simulink model "model_main5"  (R2023b)
settings: Solver=ode4  StartTime=0.0  StopTime=1000  FixedStep=dt  RelTol=1e-3
InitFcn:
  | model_init
values from neighbouring files (symbols this model uses):
  dt = 0.01    [model_init.m]
  Iws = diag([1 1 1 1])*0.2274    [model_init.m]
  m_tot = 3300    [model_init.m]
  norm_Ib = diag(diag(SC_Ib) / norm(diag(SC_Ib)))    [model_init.m]
  Omega1_init = 2000*rpm2rad    (= 209.439510239)    [model_init.m]
  Omega2_init = 2000*rpm2rad    (= 209.439510239)    [model_init.m]
  Omega3_init = 2000*rpm2rad    (= 209.439510239)    [model_init.m]
  Omega4_init = 2000*rpm2rad    (= 209.439510239)    [model_init.m]
  Omega_ref = [1000 1000 1000 1000]*rpm2rad    [model_init.m]
  port_offset = [7.196; 0 ; 0.618]    [model_init.m]
  qb0 = angle2quat(ag0(1),ag0(2),ag0(3),'ZYX')'    [model_init.m]
  rad2rpm = 1/rpm2rad    (= 9.54929658551)    [model_init.m]
  RCS_F = 1.0    (= 1)    [model_init.m]
  RCS_Pos = [RCS1_POS , RCS2_POS , RCS3_POS , RCS4_POS ,            RCS5_POS , RCS6_POS , RCS7_POS , RCS8_POS ,            RCS9_POS , RCS10_POS, RCS11_POS, RCS12_POS,            RCS13_POS, RCS14_POS, RCS15_POS, RCS16_POS]    [model_init.m]
  RCS_PWM_Freq = 0.1    [model_init.m]
  RCS_Sampling_time = 0.01    [model_init.m]
  RCS_THR_vec = [RCS1_THR , RCS2_THR , RCS3_THR , RCS4_THR,                 RCS5_THR , RCS6_THR , RCS7_THR , RCS8_THR,                 RCS9_THR , RCS10_THR, RCS11_THR, RCS12_THR,                 RCS13_THR, RCS14_THR, RCS15_THR, RCS16_THR]    [model_init.m]
  REL_port_POS_I_0 = REL_TS_POS_I_0 - quat2rotm(qb0') * port_offset    [model_init.m]
  REL_port_VEL_I_0 = REL_TS_VEL_I_0 - quat2rotm(qb0') * cross(wb0,port_offset)    [model_init.m]
  REL_TS_POS_I_0 = TS_pos0 - SC_pos0    [model_init.m]
  REL_TS_VEL_I_0 = TS_vel0 - SC_vel0    [model_init.m]
  RW_As = [RW1_Axis,RW2_Axis,RW3_Axis,RW4_Axis]    [model_init.m]
  RW_Max_Speed = 4200*rpm2rad    (= 439.822971503)    [model_init.m]
  RW_t_max = 0.5    [model_init.m]
  SC_Ib = [1843.56  -0.0019  -803.89 ... (first row only)    [model_init.m]
  SC_state0 = kepel_statvec (SC_Kepler)    [model_init.m]
  TS_Ib = diag([1 1 1])    [model_init.m]
  TS_qb0 = angle2quat(deg2rad(0),deg2rad(0),deg2rad(0),'ZYX')'    [model_init.m]
  TS_state0 = kepel_statvec (TS_Kepler)    [model_init.m]
  TS_wb0 = deg2rad([0 0 0]')    [model_init.m]
  wb0 = deg2rad([-0.3 -0.1 0.2])'    [model_init.m]
undefined symbols (not defined in the file or in its folder): RCS_F_vec, RCS_pos, SS_Total_Mass, TC_Kepler
libraries: simulink x16, simulink_extras x16, aerolibutil x9, sharedtransform x8
(part 2 of 3)

== system model_main5/PWPFM/Subsystem2 ==
  In1 : Inport
  Constant : Constant  Value=0
  Constant1 : Constant
  PWPFM_Filter2 : TransferFcn  Numerator=1  Denominator=[0.275 1]
  Schmitt_Trigger1 : Relay  OnSwitchValue=0.127  OffSwitchValue=-0.127
  Sum_PWPFM1 : Sum  Inputs=|+-
  Switch : Switch  Criteria=u2 > Threshold  Threshold=0.25  SaturateOnIntegerOverflow=off  InputSameDT=off
  Switch2 : Switch  Criteria=u2 > Threshold  Threshold=1  SaturateOnIntegerOverflow=off  InputSameDT=off
  F_gated : Outport
  wires:
  In1/1 -> Switch/2, Switch/1
  Constant/1 -> Switch/3
  Switch/1 -> Switch2/2, Switch2/3
  Constant1/1 -> Switch2/1
  Switch2/1 -> Sum_PWPFM1/1
  Schmitt_Trigger1/1 -> PWPFM_Filter2/1, F_gated/1
  Sum_PWPFM1/1 -> Schmitt_Trigger1/1
  PWPFM_Filter2/1 -> Sum_PWPFM1/2

== system model_main5/PWPFM/Subsystem3 ==
  In1 : Inport
  Constant : Constant  Value=0
  Constant1 : Constant
  PWPFM_Filter2 : TransferFcn  Numerator=1  Denominator=[0.275 1]
  Schmitt_Trigger1 : Relay  OnSwitchValue=0.127  OffSwitchValue=-0.127
  Sum_PWPFM1 : Sum  Inputs=|+-
  Switch : Switch  Criteria=u2 > Threshold  Threshold=0.25  SaturateOnIntegerOverflow=off  InputSameDT=off
  Switch2 : Switch  Criteria=u2 > Threshold  Threshold=1  SaturateOnIntegerOverflow=off  InputSameDT=off
  F_gated : Outport
  wires:
  PWPFM_Filter2/1 -> Sum_PWPFM1/2
  Sum_PWPFM1/1 -> Schmitt_Trigger1/1
  Schmitt_Trigger1/1 -> F_gated/1, PWPFM_Filter2/1
  Switch2/1 -> Sum_PWPFM1/1
  Constant1/1 -> Switch2/1
  Switch/1 -> Switch2/3, Switch2/2
  Constant/1 -> Switch/3
  In1/1 -> Switch/1, Switch/2

== system model_main5/PWPFM/Subsystem4 ==
  In1 : Inport
  Constant : Constant  Value=0
  Constant1 : Constant
  PWPFM_Filter2 : TransferFcn  Numerator=1  Denominator=[0.275 1]
  Schmitt_Trigger1 : Relay  OnSwitchValue=0.127  OffSwitchValue=-0.127
  Sum_PWPFM1 : Sum  Inputs=|+-
  Switch : Switch  Criteria=u2 > Threshold  Threshold=0.25  SaturateOnIntegerOverflow=off  InputSameDT=off
  Switch2 : Switch  Criteria=u2 > Threshold  Threshold=1  SaturateOnIntegerOverflow=off  InputSameDT=off
  F_gated : Outport
  wires:
  In1/1 -> Switch/2, Switch/1
  Constant/1 -> Switch/3
  Switch/1 -> Switch2/2, Switch2/3
  Constant1/1 -> Switch2/1
  Switch2/1 -> Sum_PWPFM1/1
  Schmitt_Trigger1/1 -> PWPFM_Filter2/1, F_gated/1
  Sum_PWPFM1/1 -> Schmitt_Trigger1/1
  PWPFM_Filter2/1 -> Sum_PWPFM1/2

== system model_main5/PWPFM/Subsystem5 ==
  In1 : Inport
  Constant : Constant  Value=0
  Constant1 : Constant
  PWPFM_Filter2 : TransferFcn  Numerator=1  Denominator=[0.275 1]
  Schmitt_Trigger1 : Relay  OnSwitchValue=0.127  OffSwitchValue=-0.127
  Sum_PWPFM1 : Sum  Inputs=|+-
  Switch : Switch  Criteria=u2 > Threshold  Threshold=0.25  SaturateOnIntegerOverflow=off  InputSameDT=off
  Switch2 : Switch  Criteria=u2 > Threshold  Threshold=1  SaturateOnIntegerOverflow=off  InputSameDT=off
  F_gated : Outport
  wires:
  PWPFM_Filter2/1 -> Sum_PWPFM1/2
  Sum_PWPFM1/1 -> Schmitt_Trigger1/1
  Schmitt_Trigger1/1 -> F_gated/1, PWPFM_Filter2/1
  Switch2/1 -> Sum_PWPFM1/1
  Constant1/1 -> Switch2/1
  Switch/1 -> Switch2/3, Switch2/2
  Constant/1 -> Switch/3
  In1/1 -> Switch/1, Switch/2

== system model_main5/PWPFM/Subsystem6 ==
  In1 : Inport
  Constant : Constant  Value=0
  Constant1 : Constant
  PWPFM_Filter2 : TransferFcn  Numerator=1  Denominator=[0.275 1]
  Schmitt_Trigger1 : Relay  OnSwitchValue=0.127  OffSwitchValue=-0.127
  Sum_PWPFM1 : Sum  Inputs=|+-
  Switch : Switch  Criteria=u2 > Threshold  Threshold=0.25  SaturateOnIntegerOverflow=off  InputSameDT=off
  Switch2 : Switch  Criteria=u2 > Threshold  Threshold=1  SaturateOnIntegerOverflow=off  InputSameDT=off
  F_gated : Outport
  wires:
  In1/1 -> Switch/2, Switch/1
  Constant/1 -> Switch/3
  Switch/1 -> Switch2/2, Switch2/3
  Constant1/1 -> Switch2/1
  Switch2/1 -> Sum_PWPFM1/1
  Schmitt_Trigger1/1 -> PWPFM_Filter2/1, F_gated/1
  Sum_PWPFM1/1 -> Schmitt_Trigger1/1
  PWPFM_Filter2/1 -> Sum_PWPFM1/2

== system model_main5/PWPFM/Subsystem7 ==
  In1 : Inport
  Constant : Constant  Value=0
  Constant1 : Constant
  PWPFM_Filter2 : TransferFcn  Numerator=1  Denominator=[0.275 1]
  Schmitt_Trigger1 : Relay  OnSwitchValue=0.127  OffSwitchValue=-0.127
  Sum_PWPFM1 : Sum  Inputs=|+-
  Switch : Switch  Criteria=u2 > Threshold  Threshold=0.25  SaturateOnIntegerOverflow=off  InputSameDT=off
  Switch2 : Switch  Criteria=u2 > Threshold  Threshold=1  SaturateOnIntegerOverflow=off  InputSameDT=off
  F_gated : Outport
  wires:
  In1/1 -> Switch/2, Switch/1
  Constant/1 -> Switch/3
  Switch/1 -> Switch2/2, Switch2/3
  Constant1/1 -> Switch2/1
  Switch2/1 -> Sum_PWPFM1/1
  Schmitt_Trigger1/1 -> PWPFM_Filter2/1, F_gated/1
  Sum_PWPFM1/1 -> Schmitt_Trigger1/1
  PWPFM_Filter2/1 -> Sum_PWPFM1/2

== system model_main5/PWPFM/Subsystem8 ==
  In1 : Inport
  Constant : Constant  Value=0
  Constant1 : Constant
  PWPFM_Filter2 : TransferFcn  Numerator=1  Denominator=[0.275 1]
  Schmitt_Trigger1 : Relay  OnSwitchValue=0.127  OffSwitchValue=-0.127
  Sum_PWPFM1 : Sum  Inputs=|+-
  Switch : Switch  Criteria=u2 > Threshold  Threshold=0.25  SaturateOnIntegerOverflow=off  InputSameDT=off
  Switch2 : Switch  Criteria=u2 > Threshold  Threshold=1  SaturateOnIntegerOverflow=off  InputSameDT=off
  F_gated : Outport
  wires:
  PWPFM_Filter2/1 -> Sum_PWPFM1/2
  Sum_PWPFM1/1 -> Schmitt_Trigger1/1
  Schmitt_Trigger1/1 -> F_gated/1, PWPFM_Filter2/1
  Switch2/1 -> Sum_PWPFM1/1
  Constant1/1 -> Switch2/1
  Switch/1 -> Switch2/3, Switch2/2
  Constant/1 -> Switch/3
  In1/1 -> Switch/1, Switch/2

== system model_main5/PWPFM/Subsystem9 ==
  In1 : Inport
  Constant : Constant  Value=0
  Constant1 : Constant
  PWPFM_Filter2 : TransferFcn  Numerator=1  Denominator=[0.275 1]
  Schmitt_Trigger1 : Relay  OnSwitchValue=0.127  OffSwitchValue=-0.127
  Sum_PWPFM1 : Sum  Inputs=|+-
  Switch : Switch  Criteria=u2 > Threshold  Threshold=0.25  SaturateOnIntegerOverflow=off  InputSameDT=off
  Switch2 : Switch  Criteria=u2 > Threshold  Threshold=1  SaturateOnIntegerOverflow=off  InputSameDT=off
  F_gated : Outport
  wires:
  In1/1 -> Switch/2, Switch/1
  Constant/1 -> Switch/3
  Switch/1 -> Switch2/2, Switch2/3
  Constant1/1 -> Switch2/1
  Switch2/1 -> Sum_PWPFM1/1
  Schmitt_Trigger1/1 -> PWPFM_Filter2/1, F_gated/1
  Sum_PWPFM1/1 -> Schmitt_Trigger1/1
  PWPFM_Filter2/1 -> Sum_PWPFM1/2

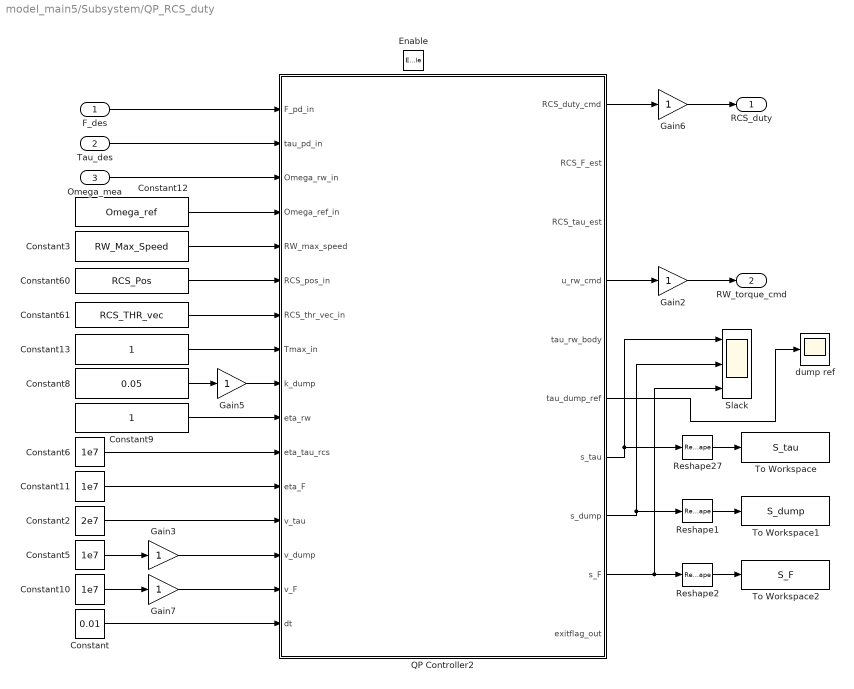
== system model_main5/Subsystem/QP_RCS_duty ==
  F_des : Inport
  Tau_des : Inport  Port=2
  Omega_mea : Inport  Port=3
  Enable : EnablePort
  Constant : Constant  Value=0.01
  Constant{5..6,10..11} (4 alike) : Constant  Value=1e7
  Constant12 : Constant  Value=Omega_ref
  Constant13 : Constant
  Constant2 : Constant  Value=2e7
  Constant3 : Constant  Value=RW_Max_Speed
  Constant60 : Constant  Value=RCS_Pos
  Constant61 : Constant  Value=RCS_THR_vec
  Constant8 : Constant  Value=0.05
  Constant9 : Constant
  Gain{2..3,5..7} (5 alike) : Gain
  QP Controller2 : MATLAB Function  TreatAsAtomicUnit=on
  Reshape1 : Reshape  OutputDimensionality=Row vector (2-D)
  Reshape2 : Reshape  OutputDimensionality=Row vector (2-D)
  Reshape27 : Reshape  OutputDimensionality=Row vector (2-D)
  Slack : Scope  NumInputPorts=3
  To Workspace : ToWorkspace  VariableName=S_tau  SampleTime=-1
  To Workspace1 : ToWorkspace  VariableName=S_dump  SampleTime=-1
  To Workspace2 : ToWorkspace  VariableName=S_F  SampleTime=-1
  dump ref : Scope
  RCS_duty : Outport
  RW_torque_cmd : Outport  Port=2
  wires:
  QP Controller2/4(u_rw_cmd) -> Gain2/1
  Tau_des/1 -> QP Controller2/2(tau_pd_in)
  Omega_mea/1 -> QP Controller2/3(Omega_rw_in)
  Constant3/1 -> QP Controller2/5(RW_max_speed)
  Constant2/1 -> QP Controller2/13(v_tau)
  Constant6/1 -> QP Controller2/11(eta_tau_rcs)
  Constant5/1 -> Gain3/1
  Constant/1 -> QP Controller2/16(dt)
  Gain2/1 -> RW_torque_cmd/1
  Gain3/1 -> QP Controller2/14(v_dump)
  Constant12/1 -> QP Controller2/4(Omega_ref_in)
  Constant8/1 -> Gain5/1
  Constant9/1 -> QP Controller2/10(eta_rw)
  Gain5/1 -> QP Controller2/9(k_dump)
  F_des/1 -> QP Controller2/1(F_pd_in)
  QP Controller2/1(RCS_duty_cmd) -> Gain6/1
  Gain6/1 -> RCS_duty/1
  Constant10/1 -> Gain7/1
  Gain7/1 -> QP Controller2/15(v_F)
  Constant11/1 -> QP Controller2/12(eta_F)
  QP Controller2/7(s_tau) -> Slack/1, Reshape27/1
  QP Controller2/8(s_dump) -> Reshape1/1, Slack/2
  QP Controller2/9(s_F) -> Reshape2/1, Slack/3
  Reshape27/1 -> To Workspace/1
  Reshape1/1 -> To Workspace1/1
  Reshape2/1 -> To Workspace2/1
  Constant61/1 -> QP Controller2/7(RCS_thr_vec_in)
  QP Controller2/6(tau_dump_ref) -> dump ref/1
  Constant13/1 -> QP Controller2/8(Tmax_in)
  Constant60/1 -> QP Controller2/6(RCS_pos_in)

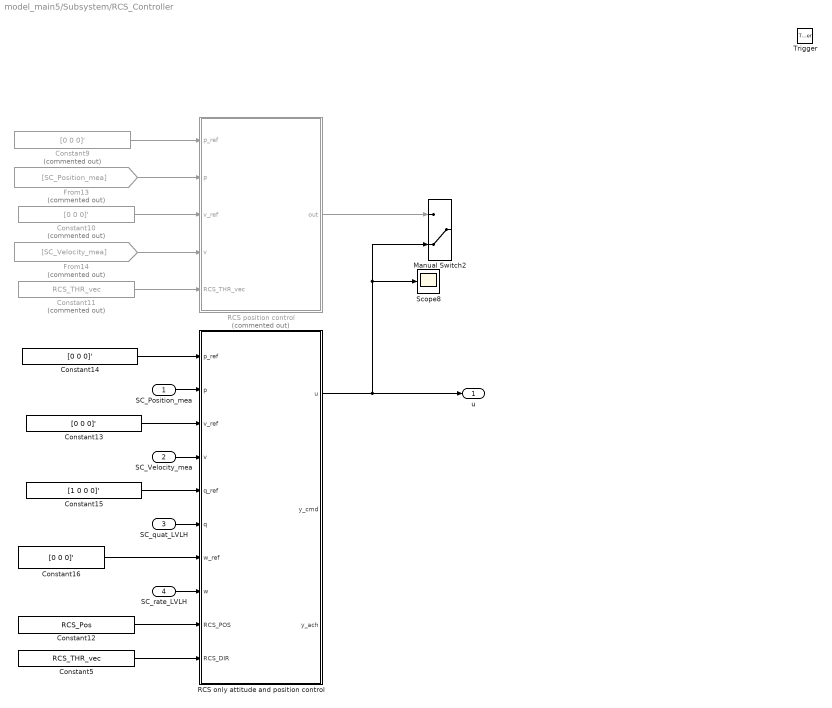
== system model_main5/Subsystem/RCS_Controller ==
  SC_Position_mea : Inport
  SC_Velocity_mea : Inport  Port=2
  SC_quat_LVLH : Inport  Port=3
  SC_rate_LVLH : Inport  Port=4
  Trigger : TriggerPort  TriggerType=either  VariantControl=(inherit)  PortDimensions=1
  Constant10 : Constant  Commented=on  Value=[0 0 0]'
  Constant11 : Constant  Commented=on  Value=RCS_THR_vec
  Constant12 : Constant  Value=RCS_Pos
  Constant13 : Constant  Value=[0 0 0]'
  Constant14 : Constant  Value=[0 0 0]'
  Constant15 : Constant  Value=[1 0 0 0]'
  Constant16 : Constant  Value=[0 0 0]'
  Constant5 : Constant  Value=RCS_THR_vec
  Constant9 : Constant  Commented=on  Value=[0 0 0]'
  From13 : From  Commented=on  GotoTag=SC_Position_mea  TagVisibility=global
  From14 : From  Commented=on  GotoTag=SC_Velocity_mea  TagVisibility=global
  Manual Switch2 : ManualSwitch  CurrentSetting=0
  RCS only attitude and position control : MATLAB Function  TreatAsAtomicUnit=on
  RCS position control : MATLAB Function  Commented=on  TreatAsAtomicUnit=on
  Scope8 : Scope
  u : Outport
  wires:
  Constant5/1 -> RCS only attitude and position control/10(RCS_DIR)
  SC_quat_LVLH/1 -> RCS only attitude and position control/6(q)
  Constant12/1 -> RCS only attitude and position control/9(RCS_POS)
  SC_rate_LVLH/1 -> RCS only attitude and position control/8(w)
  SC_Velocity_mea/1 -> RCS only attitude and position control/4(v)
  From13/1 -> RCS position control/2(p)
  RCS only attitude and position control/1(u) -> Manual Switch2/2, Scope8/1, u/1
  Constant13/1 -> RCS only attitude and position control/3(v_ref)
  Constant15/1 -> RCS only attitude and position control/5(q_ref)
  RCS position control/1(out) -> Manual Switch2/1
  Constant16/1 -> RCS only attitude and position control/7(w_ref)
  Constant10/1 -> RCS position control/3(v_ref)
  Constant9/1 -> RCS position control/1(p_ref)
  Constant11/1 -> RCS position control/5(RCS_THR_vec)
  SC_Position_mea/1 -> RCS only attitude and position control/2(p)
  Constant14/1 -> RCS only attitude and position control/1(p_ref)
  From14/1 -> RCS position control/4(v)

== matlab function model_main5/Subsystem/RCS_Controller/RCS only attitude and position control ==
  data: p_ref input; u output; p input; v_ref input; v input; q_ref input; q input; w_ref input; w input; RCS_POS input; RCS_DIR input; y_cmd output; y_ach output
function [u, y_cmd, y_ach] = fcn( ...
                                  p_ref, p, v_ref, v, ...          % position control
                                  q_ref, q, w_ref, w, ...          % attitude control (quat + body rates)
                                  RCS_POS, RCS_DIR)                % thruster geometry
%#codegen
% p, v : 3x1 [m], [m/s]
% q_ref, q : 4x1 quaternion (scalar-first: [qw qx qy qz]')
% w_ref, w : 3x1 [rad/s] (body frame)
% RCS_POS : 3xN position vectors of thrusters wrt CoM [m]
% RCS_DIR : 3xN thrust direction unit vectors [N/A] in body frame
% u : Nx1 thrust commands [N]

% ====== Parameters ======
Tmax = 22;       % [N]
m    = 2000;     % [kg]

% Translational PD gains
Kp_p = 2 * diag([1 1 1]);
Kd_p = 4 * diag([1 1 1]);

% Attitude PD gains (원하시면 사용하신 K1,K2 그대로 넣으셔도 됩니다)
Kq = 0.5 * diag([1 1 1]);    % quaternion-vector part gain
Kw = 2  * diag([1 1 1]);    % angular-rate gain

% (선택) 힘/토크 가중치: 단위/스케일 차이 때문에 보통 넣는 걸 권장합니다.
wF   = 1.0;    % force weight
wTau = 1.0;    % torque weight (필요 시 크게/작게 조정)

% ====== 1) Translation: PD -> F_cmd ======
e_p = p_ref - p;
e_v = v_ref - v;

a_cmd = Kp_p*e_p + Kd_p*e_v;
F_cmd = m * a_cmd;              % 3x1

% ====== 2) Attitude: quaternion error + rate error -> Tau_cmd ======
qe = quat_err_scalar_first(q_ref, q);     % q_err = q_ref ⊗ conj(q)
% 쿼터니언 언와인딩 방지(연속성)
if qe(1) < 0
    qe = -qe;
end
qe_v = qe(2:4);

we = w - w_ref;                 % body rate error (원하시면 w_ref-w 로 바꾸셔도 됨)

% 기본적인 PD 토크(부호는 시스템 정의에 맞게 조정 가능)
Tau_cmd = -(Kq*qe_v + Kw*we);    % 3x1

% ====== 3) Build 6xN allocation matrix B ======
N = size(RCS_DIR, 2);

B = zeros(6, N);
for i = 1:N
    ti = RCS_DIR(:, i);          % 3x1
    ri = RCS_POS(:, i);          % 3x1
    B(1:3, i) = ti;
    B(4:6, i) = cross(ri, ti);
end

% ====== 4) Stack command y = [F; Tau] and solve allocation ======
y_cmd = [wF*F_cmd; wTau*Tau_cmd];      % 6x1
Bw    = [wF*B(1:3,:); wTau*B(4:6,:)];  % weighted B

% 간단 대안: pinv + clip + active-set 반복(툴박스 없이 가능)
u = rcs_allocate_pinv_clip_iter(Bw, y_cmd, Tmax);

y_ach = B*u;    % achieved (unweighted, physical)

end

% ===== Helper: iterative clipped pseudo-inverse allocation =====
function u = rcs_allocate_pinv_clip_iter(B, y, Tmax)
%#codegen
N = size(B,2);

% 초기 해
u = pinv(B) * y;

% active-set 반복: 0 또는 Tmax에 걸린 추력기는 고정하고 나머지만 재해결
MAX_IT = 10;
for k = 1:MAX_IT
    u_prev = u;

    % bounds 적용
    u = max(u, 0);
    u = min(u, Tmax);

    % 자유 변수 마스크
    free = (u > 1e-9) & (u < Tmax - 1e-9);

    if ~any(free)
        break;
    end

    % 고정된 변수 기여를 빼고, 자유 변수만 재계산
    y_res = y - B(:, ~free) * u(~free);
    Bf    = B(:, free);

    uf = pinv(Bf) * y_res;

    u(free) = uf;

    % 수렴 체크
    if norm(u - u_prev) < 1e-6
        break;
    end
end
end

% ===== Helper: quaternion error (scalar-first) =====
function qe = quat_err_scalar_first(q_ref, q)
%#codegen
% qe = q_ref ⊗ conj(q)
qc = [q(1); -q(2); -q(3); -q(4)];

qe = quat_mul_scalar_first(q_ref, qc);
end

function q = quat_mul_scalar_first(q1, q2)
%#codegen
w1=q1(1); x1=q1(2); y1=q1(3); z1=q1(4);
w2=q2(1); x2=q2(2); y2=q2(3); z2=q2(4);

q = [ ...
    w1*w2 - x1*x2 - y1*y2 - z1*z2; ...
    w1*x2 + x1*w2 + y1*z2 - z1*y2; ...
    w1*y2 - x1*z2 + y1*w2 + z1*x2; ...
    w1*z2 + x1*y2 - y1*x2 + z1*w2  ...
    ];
end

== matlab function model_main5/Subsystem/RCS_Controller/RCS position control ==
  data: p_ref input; out output; p input; v_ref input; v input; RCS_THR_vec input
function out = fcn(p_ref, p, v_ref, v, RCS_THR_vec)
% ====== 파라미터 ======
Tmax   = 22;       % [N]
m = 2000;
% pwmMax = 65535;    % 예: 16-bit
% pwmMin = 0;        % 필요하면 최소 구동값 넣기
Kp = 20*diag([1 1 1]);
Kd = 40*diag([1 1 1]);
% ====== 1) PD -> F_cmd ======
e_p = p_ref - p;
e_v = v_ref - v;

a_cmd = Kp*e_p + Kd*e_v;
F_cmd = m * a_cmd;

% ====== 2) Allocation ======
% [u, F_ach] = rcs_allocate_lsqlin(F_cmd, RCS_THR_vec, Tmax); % toolbox 권장
[u, F_ach] = rcs_allocate_pinv_clip(F_cmd, RCS_THR_vec, Tmax); % 간단 대안

% ====== 3) PWM ======
% pwm = thrust_to_pwm(u, Tmax, pwmMax, pwmMin);
out = u./1;
% (디버그)
% disp("F_cmd  = " + mat2str(F_cmd',4))
% disp("F_ach  = " + mat2str(F_ach',4))
% disp("u(N)   = " + mat2str(u',4))
% disp("pwm    = " + mat2str(pwm',4))

end

function [u, F_ach] = rcs_allocate_pinv_clip(F_cmd, RCS_THR_vec, Tmax)
    B = RCS_THR_vec;     % 3xN
    u = pinv(B) * F_cmd; % unconstrained

    % Thruster는 보통 단방향(0~Tmax)이므로 음수는 0으로
    u = max(u, 0);
    u = min(u, Tmax);

    F_ach = B*u;
end


function pwm = thrust_to_pwm(u, Tmax, pwmMax, pwmMin)
    % u: Nx1 thrust command [N]
    % pwmMax: 예) 65535 또는 255
    % pwmMin: (선택) 밸브/드라이버가 실제로 열리는 최소 duty가 있으면 반영

    duty = u(:) / Tmax;          % 0~1
    duty = max(0, min(1, duty));

    if nargin >= 4 && pwmMin > 0
        % duty>0인 경우에만 최소 구동 듀티 적용(데드존)
        duty(duty>0) = max(duty(duty>0), pwmMin/pwmMax);
    end

    pwm = round(duty * pwmMax);
end

== matlab function model_main5/Subsystem/Attitude_PD_control1 ==
  settings: updateMethod=DISCRETE
  data: F_B_cmd output; r_I input; v_I input; q_IB input; r_d input; v_d input; a_d input; m input
function F_B_cmd  = CTRL_WRENCH_6DOF(r_I, v_I, q_IB, r_d, v_d, a_d, m)
%#codegen
% ============================================================
% Controller block
% Input :
%   r_I      [3x1] current position in inertial frame
%   v_I      [3x1] current velocity in inertial frame
%   q_IB     [4x1] quaternion [qw qx qy qz], Body -> Inertial
%   omega_B  [3x1] current angular velocity in body frame
%
%   r_d      [3x1] desired position in inertial frame
%   v_d      [3x1] desired velocity in inertial frame
%   a_d      [3x1] desired acceleration in inertial frame
%   q_d      [4x1] desired quaternion, Body -> Inertial
%   omega_d_B[3x1] desired angular velocity in body frame
%
%   m        scalar mass
%   J        [3x3] inertia matrix in body frame
%
% Output:
%   F_B_cmd    [3x1] desired total body force
%   tau_B_cmd  [3x1] desired total body torque
% ============================================================

    % -------------------------
    % Quaternion normalize
    % -------------------------
    q_IB = quat_normalize(q_IB); 

    % -------------------------
    % Gains (example)
    % -------------------------
    Kp_r = 10*diag([0.01, 0.006, 0.006]);   % position gain
    Kd_r = 100*diag([0.01, 0.01, 0.01]);   % velocity damping
 
    % Kp_r = diag([0.010, 0.010, 0.010]);   % position gain
    % Kd_r = diag([0.060, 0.060, 0.060]);   % velocity damping

    % -------------------------
    % Position control
    % inertial acceleration command
    % -------------------------
    e_r = r_I - r_d;
    e_v = v_I - v_d;

    a_cmd   = a_d - Kp_r * e_r - Kd_r * e_v;
    F_I_cmd = m * a_cmd;

    % Convert inertial force -> body force
    R_IB    = quat_to_rotm(q_IB);
    F_B_cmd = R_IB.' * F_I_cmd;
 
end


% ============================================================
% Local helper functions
% ============================================================

function qn = quat_normalize(q)
    n = norm(q);
    if n < 1e-12
        qn = [1;0;0;0];
    else
        qn = q / n;
    end
end
 

function R = quat_to_rotm(q)
    % q = [qw qx qy qz], Body -> Inertial
    qw = q(1); qx = q(2); qy = q(3); qz = q(4);

    R = [1-2*(qy^2+qz^2),   2*(qx*qy-qz*qw),   2*(qx*qz+qy*qw);
         2*(qx*qy+qz*qw),   1-2*(qx^2+qz^2),   2*(qy*qz-qx*qw);
         2*(qx*qz-qy*qw),   2*(qy*qz+qx*qw),   1-2*(qx^2+qy^2)];
end

== matlab function model_main5/Subsystem/Thruster Allocation ==
  settings: updateMethod=DISCRETE
  data: u_pwm output; F_B_cmd input; tau_B_cmd input; F_B_real output; tau_B_real output; r input; d input; F_max input
function [u_pwm, F_B_real, tau_B_real] = ALLOC_THRUSTER_PWM_16(F_B_cmd, tau_B_cmd, r, d, F_max)
%#codegen
% ============================================================
% Allocation block
% Input :
%   F_B_cmd    [3x1] desired total body force
%   tau_B_cmd  [3x1] desired total body torque
%
% Output:
%   u_pwm      [12x1] thruster duty command, 0 ~ 1
%   F_B_real   [3x1] realized body force after allocation
%   tau_B_real [3x1] realized body torque after allocation
%
% Example:
%   12-thruster layout for 6DoF control
%   Replace thruster geometry / Tmax below with your real spacecraft values.
% ============================================================

    % Build 6x12 thruster mapping matrix A
    A = build_thruster_matrix( 16, r, d, F_max);

    % Desired wrench
    w_cmd = [F_B_cmd; tau_B_cmd];

    % Bounded least-squares allocation: 0 <= u <= 1
    u_pwm = bounded_allocator_0_1(A, w_cmd);

    % Realized wrench
    w_real     = A * u_pwm;
    F_B_real   = w_real(1:3);
    tau_B_real = w_real(4:6);
end


% ============================================================
% Thruster layout
% ============================================================
function A = build_thruster_matrix(N, r, d, F_max)
    % --------------------------------------------------------
    % Example spacecraft half-size [m]
    % Replace with your real geometry
    % --------------------------------------------------------
    % L = 0.50;   % lever arm

    % --------------------------------------------------------
    % Max thrust of each thruster [N]
    % Replace with your real thruster max force
    % --------------------------------------------------------
    Tmax = F_max * ones(N,1);

    % --------------------------------------------------------
    % Thruster positions r_i in body frame [m]
    % Each column is one thruster position
    % --------------------------------------------------------
    % r = [ ...
    %      0,   0,   0,   0,   L,  -L,   L,  -L,   L,  -L,   L,  -L;
    %      L,  -L,   L,  -L,   0,   0,   0,   0,   L,   L,  -L,  -L;
    %      L,  -L,  -L,   L,   L,  -L,  -L,   L,   0,   0,   0,   0 ];

    % --------------------------------------------------------
    % Thruster unit directions d_i in body frame
    %
    % T1,T2 : +X
    % T3,T4 : -X
    % T5,T6 : +Y
    % T7,T8 : -Y
    % T9,T10: +Z
    % T11,T12:-Z
    % --------------------------------------------------------
    % d = [ ...
    %      1,   1,  -1,  -1,   0,   0,   0,   0,   0,   0,   0,   0;
    %      0,   0,   0,   0,   1,   1,  -1,  -1,   0,   0,   0,   0;
    %      0,   0,   0,   0,   0,   0,   0,   0,   1,   1,  -1,  -1 ];

    % --------------------------------------------------------
    % Build A = [F; tau], size 6x12
    % --------------------------------------------------------
    A = zeros(6,N);

    for i = 1:N
        f_i       = Tmax(i) * d(:,i);
        tau_i     = cross(r(:,i), f_i);
        A(:,i)    = [f_i; tau_i];
    end
end


% ============================================================
% Bounded allocator: 0 <= u <= 1
% Codegen-friendly fixed-size active-set style
% ============================================================
function u = bounded_allocator_0_1(A, w_cmd)
    N = 16;
    u = zeros(N,1);

    % free_mask(i)=true means this thruster is still free to solve
    free_mask = true(N,1);

    lambda = 1e-8;   % small damping

    for iter = 1:(N+1)

        % Residual after fixed/saturated thrusters
        w_res = w_cmd;
        for i = 1:N
            if ~free_mask(i)
                w_res = w_res - A(:,i) * u(i);
            end
        end

        % Collect free columns into Af (fixed-size construction)
        Af  = zeros(6,N);
        idx = zeros(N,1);
        nf  = 0;

        for i = 1:N
            if free_mask(i)
                nf = nf + 1;
                idx(nf) = i;
                Af(:,nf) = A(:,i);
            end
        end

        if nf == 0
            break;
        end

        % Minimum-norm damped solution on free set
        M       = Af * Af.' + lambda * eye(6);
        uf_full = Af.' * (M \ w_res);   % size Nx1, only first nf entries used

        % Put candidate solution into u
        for k = 1:nf
            i = idx(k);
            u(i) = uf_full(k);
        end

        % Check bounds and fix saturated variables
        violated = false;
        for k = 1:nf
            i = idx(k);

            if u(i) < 0
                u(i) = 0;
                free_mask(i) = false;
                violated = true;

            elseif u(i) > 1
                u(i) = 1;
                free_mask(i) = false;
                violated = true;
            end
        end

        if ~violated
            break;
        end
    end

    % Final clipping
    for i = 1:N
        if u(i) < 0
            u(i) = 0;
        elseif u(i) > 1
            u(i) = 1;
        end
    end
end

== matlab function model_main5/saturation ==
  data: max_speed input; res output; Omega_mea input; torque_cmd input
function res  = saturation(max_speed, Omega_mea, torque_cmd)

Omega1_mea = Omega_mea(1);
Omega2_mea = Omega_mea(2);
Omega3_mea = Omega_mea(3);
Omega4_mea = Omega_mea(4);

if abs(Omega1_mea)> max_speed
    res1 = 0;
else
    res1 = torque_cmd(1);
end

if abs(Omega2_mea)>max_speed
    res2 = 0;
else
    res2 = torque_cmd(2);
end

if abs(Omega3_mea)>max_speed
    res3 = 0;
else
    res3 = torque_cmd(3);
end

if abs(Omega4_mea)>max_speed
    res4 = 0;
else
    res4 = torque_cmd(4);
end

res = [res1,res2,res3,res4]';

end

== matlab function model_main5/TS 6-DOF Dynamics ==
  data: w input; x input; Ib input; wd output; T_ext input; F_ext input; xd output
function [wd, xd]  = eq_propagate(w, x, Ib, T_ext, F_ext)
% % 
% 출력 1: 위성 동체 좌표계 각가속도
% 출력 2: 관성좌표계 선가속도

%% Rotational Motion
% wd = [0 0 0]';
wd = inv(Ib)*(T_ext - cross(w, Ib*w));

%% Translational Motion
 
u  =  3.986004418e14; % earth gravitional parameter
Re = 6378137;      % earth radius [m]

xd = zeros(size(x));

v1_i = x(4); % x1 = dx/dt
v2_i = x(5); % y1 = dy/dt
v3_i = x(6); % z1 = dz/dt
p1_i = x(1); % x
p2_i = x(2); % y
p3_i = x(3); % z

r=sqrt(p1_i^2+p2_i^2+p3_i^2);

% % %   Keplar Motion Equatnion
% % %  => r_dd + u/(r^3)r_ = 0 => r_dd = -u/(r^3)r_
xd(1) = v1_i;
xd(2) = v2_i;
xd(3) = v3_i;
xd(4) = -u*p1_i/(r^3) +  F_ext(1);
xd(5) = -u*p2_i/(r^3) +  F_ext(2);
xd(6) = -u*p3_i/(r^3) +  F_ext(3);

end

== matlab function model_main5/Subsystem/Attitude_PD_control2 ==
  settings: updateMethod=DISCRETE
  data: q_err input; omega_B input; omega_d_B input; J input; tau_B_cmd output
function tau_B_cmd  = CTRL_WRENCH_6DOF(q_err, omega_B, omega_d_B, J)
%#codegen
% ============================================================
% Controller block
% Input :
%   r_I      [3x1] current position in inertial frame
%   v_I      [3x1] current velocity in inertial frame
%   q_IB     [4x1] quaternion [qw qx qy qz], Body -> Inertial
%   omega_B  [3x1] current angular velocity in body frame
%
%   r_d      [3x1] desired position in inertial frame
%   v_d      [3x1] desired velocity in inertial frame
%   a_d      [3x1] desired acceleration in inertial frame
%   q_d      [4x1] desired quaternion, Body -> Inertial
%   omega_d_B[3x1] desired angular velocity in body frame
%
%   m        scalar mass
%   J        [3x3] inertia matrix in body frame
%
% Output:
%   F_B_cmd    [3x1] desired total body force
%   tau_B_cmd  [3x1] desired total body torque
% ============================================================
 
    % -------------------------
    % Gains (example)
    % -------------------------
    Kq   = J*diag([0.3, 0.3, 0.3]);   % attitude gain
    Kw   = J*diag([5, 5, 5]);   % angular-rate damping

    % Kq   = diag([10.0, 10.0, 10.0]);   % attitude gain
    % Kw   = diag([6.0,  6.0,  6.0 ]);   % angular-rate damping
    % -------------------------
 
    % -------------------------
    % Attitude control 
    % -------------------------
 
    % shortest-path quaternion
    if q_err(1) < 0
        q_err = -q_err;
    end

    e_w = omega_B - omega_d_B;

    % PD + gyro compensation
    tau_B_cmd = -Kq * q_err(2:4) ...
                -Kw * e_w ...
                +cross(omega_B, J * omega_B);
end


% ============================================================
% Local helper functions
% ============================================================

function qn = quat_normalize(q)
    n = norm(q);
    if n < 1e-12
        qn = [1;0;0;0];
    else
        qn = q / n;
    end
end

function qc = quat_conj(q)
    qc = [q(1); -q(2); -q(3); -q(4)];
end

function q = quat_mul(q1, q2)
    % Hamilton product
    w1 = q1(1); x1 = q1(2); y1 = q1(3); z1 = q1(4);
    w2 = q2(1); x2 = q2(2); y2 = q2(3); z2 = q2(4);

    q = [ w1*w2 - x1*x2 - y1*y2 - z1*z2;
          w1*x2 + x1*w2 + y1*z2 - z1*y2;
          w1*y2 - x1*z2 + y1*w2 + z1*x2;
          w1*z2 + x1*y2 - y1*x2 + z1*w2 ];
end

== matlab function model_main5/Position&Attitude_PD_Controller ==
  settings: updateMethod=DISCRETE
  data: r_rel input; v_rel input; r_ref input; v_ref input; a_ref input; q input; q_err input; w_err input; wb input; F_cmd_B output; tau_cmd_B output; m_sc input; Ib input; Omega input; Kp_pos input; Kd_pos input; Kp_att input; Kd_att input; r_err output; v_err output; q output; q_err output; w_err output; a_cmd output
function [F_cmd_B, tau_cmd_B, r_err, v_err, q, q_err, w_err, a_cmd] = ...
    relative_position_los_controller( ...
    r_rel, v_rel, ...          % [3x1] relative position/velocity
    r_ref, v_ref, a_ref, ...   % [3x1] desired relative pos/vel/acc
    q, q_err, w_err, wb, m_sc, Ib,Omega, Kp_pos, Kd_pos, Kp_att, Kd_att)
 
% q, q_los_ref : scalar-first quaternion [qw qx qy qz]'
%                body -> reference
% r_rel, r_ref, v_rel, v_ref, a_ref : reference frame 기준
%
% 출력:
% F_cmd_B   : [3x1] body frame force command
% tau_cmd_B : [3x1] body frame torque command

F_cmd_B   = zeros(3,1);
tau_cmd_B = zeros(3,1);
r_err     = zeros(3,1);
v_err     = zeros(3,1);
q_err_vec = zeros(3,1);
% w_err     = zeros(3,1);
a_cmd     = zeros(3,1);

As = [ 0.70710678,  0.0,        -0.70710678,  0.0;
       0.0,         0.70710678,  0.0,        -0.70710678;
       0.70710678,  0.70710678,  0.70710678,  0.70710678 ];

% wheel spin inertias [kg*m^2]
Iws = diag([1 1 1 1])*0.227;

RW_h = As*Iws*Omega;

%% 1) Relative position controller
r_ref = quat_to_dcm_sf(q) * r_ref;
r_err = r_ref - r_rel;
v_ref = quat_to_dcm_sf(q) * cross(wb, r_ref);
v_err =  v_ref - v_rel; 

a_cmd = a_ref + Kp_pos * r_err + Kd_pos * v_err;
F_cmd_R = m_sc * a_cmd;

%% 2) Reference frame -> body frame
% q : body -> reference
% therefore F_B = C_BR' * F_R
C_BR   = quat_to_dcm_sf(q);
F_cmd_B = C_BR' * F_cmd_R;

%% 3) attitude controller
 
% shortest path
if q_err(1) < 0
    q_err = -q_err;
end

q_err_vec = q_err(2:4);

tau_cmd_B =  Kp_att * q_err_vec + Kd_att * w_err + cross(wb, Ib*wb + RW_h);  
end


function q_out = quat_mul_sf(a, b)
% scalar-first quaternion multiplication
q_out = [ a(1)*b(1) - a(2)*b(2) - a(3)*b(3) - a(4)*b(4);
    a(1)*b(2) + a(2)*b(1) + a(3)*b(4) - a(4)*b(3);
    a(1)*b(3) - a(2)*b(4) + a(3)*b(1) + a(4)*b(2);
    a(1)*b(4) + a(2)*b(3) - a(3)*b(2) + a(4)*b(1) ];
end


function C = quat_to_dcm_sf(q)
% scalar-first quaternion, body -> reference
q = q / (sqrt(sum(q.^2)) + 1e-12);

qw = q(1);
qx = q(2);
qy = q(3);
qz = q(4);

C = [1-2*(qy*qy+qz*qz),   2*(qx*qy-qw*qz),   2*(qx*qz+qw*qy);
    2*(qx*qy+qw*qz),     1-2*(qx*qx+qz*qz), 2*(qy*qz-qw*qx);
    2*(qx*qz-qw*qy),     2*(qy*qz+qw*qx),   1-2*(qx*qx+qy*qy)];
end

== matlab function model_main5/RCS_Force_Torque_Allocation ==
  settings: updateMethod=DISCRETE
  data: F_cmd input; tau_cmd input; RCS_pos input; RCS_F_vec input; Fmax input; duty output; F_est output; tau_est output; F_err output; tau_err output; sat_ratio output; wF input; wT input
function [duty, F_est, tau_est, F_err, tau_err, sat_ratio] = ...
    rcs_force_torque_allocator(F_cmd, tau_cmd, RCS_pos, RCS_F_vec, Fmax, wF, wT)

% F_cmd      : [3x1] commanded force in body frame [N]
% tau_cmd    : [3x1] commanded torque in body frame [N*m]
% RCS_pos    : [3xN] thruster positions in body frame [m]
% RCS_F_vec  : [3xN] thruster direction vectors
% wF         : scalar, force tracking weight
% wT         : scalar, torque tracking weight
%
% duty       : [N x 1], 0~1
% F_est      : [3x1], achieved force [N]
% tau_est    : [3x1], achieved torque [N*m]
% F_err      : [3x1], force error [N]
% tau_err    : [3x1], torque error [N*m]
% sat_ratio  : saturated thruster ratio

    N = size(RCS_pos, 2);

    duty      = zeros(N,1);
    F_est     = zeros(3,1);
    tau_est   = zeros(3,1);
    F_err     = zeros(3,1);
    tau_err   = zeros(3,1);
    sat_ratio = 0;

    Fmat = zeros(3, N);
    Tmat = zeros(3, N);

    for i = 1:N
        dir_i = RCS_F_vec(:,i);
        nrm   = sqrt(sum(dir_i.^2));

        if nrm > 1e-12
            dir_i = dir_i / nrm;
        else
            dir_i = [0;0;0];
        end

        Fi = Fmax * dir_i;
        Ti = cross3(RCS_pos(:,i), Fi);

        Fmat(:,i) = Fi;
        Tmat(:,i) = Ti;
    end

    % Solve:
    % min || wF*(Fmat*u - F_cmd) ||^2 + || wT*(Tmat*u - tau_cmd) ||^2
    % s.t. 0 <= u <= 1

    A = [wF * Fmat;
         wT * Tmat];

    b = [wF * F_cmd;
         wT * tau_cmd];

    H = A' * A + 1e-8 * eye(N);
    g = A' * b;

    alpha = 1.0 / (trace(H) + 1e-9);
    u = zeros(N,1);

    for k = 1:150
        grad = H * u - g;
        u    = u - alpha * grad;

        for j = 1:N
            if u(j) < 0
                u(j) = 0;
            elseif u(j) > 1
                u(j) = 1;
            end
        end
    end

    duty    = u;
    F_est   = Fmat * duty;
    tau_est = Tmat * duty;

    F_err   = F_cmd   - F_est;
    tau_err = tau_cmd - tau_est;

    sat_ratio = sum(duty > 0.999) / N;
end


function c = cross3(a, b)
    c = [ a(2)*b(3) - a(3)*b(2);
          a(3)*b(1) - a(1)*b(3);
          a(1)*b(2) - a(2)*b(1) ];
end

== matlab function model_main5/Mission_Supporter ==
  settings: updateMethod=DISCRETE
  data: rel_pos input; stop output; rel_pos_B output; rel_vel_B output; rel_angle_B output; rel_vel input; ts_q input; ts_wb input; q input; wb input; rel_w_B output
function [stop, rel_pos_B, rel_vel_B, rel_angle_B, rel_w_B] = ...
    IDSS_Stop_Check(rel_pos, rel_vel, ts_q, ts_wb, q, wb)
 
% rel_pos : TS_port_I - SS_port_I [m]
% rel_vel : TS_port_vel_I - SS_port_vel_I [m/s]
% ts_q    : target body -> ECI quaternion [qw qx qy qz]'
% ts_wb   : target angular velocity in target body frame [rad/s]
% q       : chaser body -> ECI quaternion [qw qx qy qz]'
% wb      : chaser angular velocity in chaser body frame [rad/s]
%
% 기준:
% chaser docking port 기준 +x = 1 m 위치에 target docking port 존재

%% DCM
C_TI = quat_to_dcm_sf(ts_q);  % target body -> ECI
C_SI = quat_to_dcm_sf(q);     % chaser body -> ECI

%% Relative position/velocity in chaser body frame
% rel_pos = target - chaser
rel_pos_B = C_SI' * rel_pos;

% rotating chaser body frame에서 본 상대속도
rel_vel_B = C_SI' * rel_vel - cross(wb, rel_pos_B);

%% Relative angular rate in chaser body frame
% target angular velocity expressed in ECI
w_T_I = C_TI * ts_wb;

% chaser angular velocity expressed in ECI
w_S_I = C_SI * wb;

% target relative angular velocity w.r.t. chaser, expressed in chaser body frame
rel_w_B = C_SI' * (w_T_I - w_S_I);

%% Relative attitude misalignment
% target body expressed in chaser body frame
C_ST = C_SI' * C_TI;

% rotation-vector error from C_ST
rot_vec = rotm_to_rotvec(C_ST);

% roll: x-axis, pitch/yaw: y,z-axis
roll_mis = abs(rot_vec(1));                         % [rad]
pitch_yaw_mis = sqrt(rot_vec(2)^2 + rot_vec(3)^2);  % [rad]

q_err = quatmultiply(quatinv(ts_q'), q');

if q_err(1) < 0
    q_err = -q_err;   % shortest rotation
end

eul_zyx = quat2eul(q_err, 'ZYX') ;  % [yaw_z pitch_y roll_x]
rel_angle_B = [eul_zyx(3); eul_zyx(2); eul_zyx(1)];
%% IDSS-type quantities

% 사용자가 추가한 axial position 종료점
x_ref = 1.0;       % [m]

% closing axial rate
% rel_pos_B(1)이 20 -> 1로 감소하면 rel_vel_B(1) < 0
% 따라서 closing rate는 -rel_vel_B(1)
closing_rate = -rel_vel_B(1);   % [m/s]

% lateral misalignment
lat_mis = sqrt(rel_pos_B(2)^2 + rel_pos_B(3)^2);  % [m]
 
% IDSS note 반영: pitch/yaw rate에 의한 lateral rate 성분 고려
% 접촉점/도킹축 방향 거리 x_ref에서 angular-rate-induced lateral velocity 근사
v_ang_B = cross(rel_w_B, [x_ref; 0; 0]);
lat_rate = sqrt((rel_vel_B(2) + v_ang_B(2))^2 + ...
                (rel_vel_B(3) + v_ang_B(3))^2);

% angular rates
roll_rate = abs(rel_w_B(1));                         % [rad/s]
pitch_yaw_rate = sqrt(rel_w_B(2)^2 + rel_w_B(3)^2);  % [rad/s]

%% Initial contact table
closing_min = 0.05;             % [m/s]
closing_max = 0.10;             % [m/s]
lat_rate_max = 0.04;            % [m/s]

pitch_yaw_rate_max = deg2rad(0.20);  % [rad/s]
roll_rate_max      = deg2rad(0.20);  % [rad/s]

lat_mis_max        = 0.10;                 % [m]
pitch_yaw_mis_max  = deg2rad(4.0);   % [rad]
roll_mis_max       = deg2rad(4.0);   % [rad]

%% Conditions
cond_x = (rel_pos_B(1)  <= x_ref);

cond_closing = (closing_rate <= closing_max);

cond_lat_rate = (lat_rate <= lat_rate_max);

cond_ang_rate = (pitch_yaw_rate <= pitch_yaw_rate_max) && ...
                (roll_rate <= roll_rate_max);

cond_mis = (lat_mis <= lat_mis_max) && ...
           (pitch_yaw_mis <= pitch_yaw_mis_max) && ...
           (roll_mis <= roll_mis_max);

if cond_x && cond_closing && cond_lat_rate && cond_ang_rate && cond_mis
    stop = 1;
else
    stop = 0;
end

end


function C = quat_to_dcm_sf(q)
% scalar-first quaternion, body -> ECI

q = q / (sqrt(sum(q.^2)) + 1e-12);

qw = q(1);
qx = q(2);
qy = q(3);
qz = q(4);

C = [1-2*(qy*qy+qz*qz),   2*(qx*qy-qw*qz),   2*(qx*qz+qw*qy);
     2*(qx*qy+qw*qz),     1-2*(qx*qx+qz*qz), 2*(qy*qz-qw*qx);
     2*(qx*qz-qw*qy),     2*(qy*qz+qw*qx),   1-2*(qx*qx+qy*qy)];
end


function rot_vec = rotm_to_rotvec(R)
% rotation matrix -> rotation vector
% small-angle and general-angle compatible

tr = trace(R);
cos_theta = 0.5 * (tr - 1.0);

if cos_theta > 1.0
    cos_theta = 1.0;
elseif cos_theta < -1.0
    cos_theta = -1.0;
end

theta = acos(cos_theta);

if theta < 1e-8
    rot_vec = 0.5 * [R(3,2)-R(2,3);
                     R(1,3)-R(3,1);
                     R(2,1)-R(1,2)];
else
    rot_vec = theta/(2.0*sin(theta)) * ...
              [R(3,2)-R(2,3);
               R(1,3)-R(3,1);
               R(2,1)-R(1,2)];
end

end

== matlab function model_main5/Get LOS Quaternion ==
  data: r_rel input; q output; ang_deg output; axis_rot output
function [q, ang_deg, axis_rot] = boresight_to_target_quat(r_rel)
%#codegen
% ============================================================
% boresight_to_target_quat
%
% Input:
%   r_rel    [3x1] : relative position vector
%
% Output:
%   q        [4x1] : quaternion [w; x; y; z]
%                    rotating boresight [1;0;0] to r_rel direction
%   ang_deg  [1x1] : rotation angle in degrees
%   axis_rot [3x1] : rotation axis (unit vector)
%
% Notes:
%   - boresight reference is fixed as [1; 0; 0]
%   - quaternion is scalar-first
%   - handles parallel / anti-parallel edge cases
% ============================================================

    % Reference boresight
    b_ref = [1; 0; 0];

    % Small threshold
    eps_val = 1e-12;

    % Check input norm
    r_norm = norm(r_rel);
    if r_norm < eps_val
        % Undefined direction
        q = [1; 0; 0; 0];
        ang_deg = 0;
        axis_rot = [1; 0; 0];
        return;
    end

    % Normalize target direction
    v = r_rel / r_norm;
    u = b_ref;

    % Dot product
    c = dot(u, v);
    c = max(min(c, 1.0), -1.0);   % numerical safety

    % Case 1: same direction
    if c > 1 - 1e-10
        q = [1; 0; 0; 0];
        ang_deg = 0;
        axis_rot = [1; 0; 0];
        return;
    end

    % Case 2: opposite direction
    if c < -1 + 1e-10
        % Need 180 deg rotation about any axis orthogonal to [1;0;0]
        % Choose y-axis
        axis_rot = [0; 1; 0];
        q = [0; axis_rot];   % cos(pi/2)=0, sin(pi/2)=1
        ang_deg = 180;
        return;
    end

    % General case
    cross_uv = cross(u, v);

    % Robust quaternion from two vectors:
    % q = [1 + dot(u,v); cross(u,v)] then normalize
    q = [1 + c;
         cross_uv(1);
         cross_uv(2);
         cross_uv(3)];

    q = q / norm(q);

    % Rotation angle
    ang_rad = 2 * acos(q(1));
    ang_deg = ang_rad * 180 / pi;

    % Rotation axis
    s = sqrt(1 - q(1)^2);
    if s < 1e-10
        axis_rot = [1; 0; 0];
    else
        axis_rot = q(2:4) / s;
    end
end

== matlab function model_main5/Enabled Subsystem/QP Controller ==
  settings: updateMethod=DISCRETE
  data: tau_pd input; u_rw_cmd output; Omega_rw input; RW_max_speed input; tau_rcs_max input; eta_rcs input; v1 input; v2 input; dt input; tau_rcs_cmd output; tau_rw_body output; tau_dump_ref output; s1 output; s2 output; exitflag_out output
function [u_rw_cmd, tau_rcs_cmd, tau_rw_body, tau_dump_ref, s1, s2, exitflag_out] = ...
    QP_Controller(tau_pd, Omega_rw, RW_max_speed, tau_rcs_max, eta_rcs, v1, v2, dt)
 
% QP with two slack variables:
%   s1 : attitude torque slack
%   s2 : dumping torque slack
%
% Inputs
%   tau_pd       [3x1] desired total body torque from PD [N*m]
%   Omega_rw     [4x1] current wheel speeds [rad/s]
%   RW_max_speed [1x1] wheel speed limit [rad/s]
%   tau_rcs_max  [3x1] approximate RCS body torque bound [N*m]
%   eta_rcs      [1x1] RCS effort weight
%   v1           [1x1] attitude slack weight
%   v2           [1x1] dumping slack weight
%   dt           [1x1] sample time [s]
%
% Outputs
%   u_rw_cmd     [4x1] RW wheel torque command [N*m]
%   tau_rcs_cmd  [3x1] RCS dumping body torque command [N*m]
%   tau_rw_body  [3x1] RW body torque [N*m]
%   tau_dump_ref [3x1] desired dumping torque reference [N*m]
%   s1           [3x1] attitude torque slack [N*m]
%   s2           [3x1] dumping torque slack [N*m]
%   exitflag_out [1x1] quadprog exitflag

persistent u_save;

if isempty(u_save)
    u_save = zeros(13,1);
end
 
u_prev   = u_save;

tau_pd      = reshape(tau_pd,      [3,1]);
Omega_rw    = reshape(Omega_rw,    [4,1]);
tau_rcs_max = reshape(tau_rcs_max, [3,1]);
Omega_ref = 1000 * pi/30 * ones(4,1);

%% RW geometry from current model
% tau_rw_body = -As * u_rw_cmd
As = [ 0.70710678,  0.0,        -0.70710678,  0.0;
       0.0,         0.70710678,  0.0,        -0.70710678;
       0.70710678,  0.70710678,  0.70710678,  0.70710678 ];

Iws = 0.227 * eye(4);

%% wheel limits
% Wheel torque limits [N*m]
u_rw_max = 0.5 * ones(4,1);
u_rw_min = -u_rw_max;

% Wheel torque rate limits [N*m/s]
du_max = [0.50; 0.50; 0.50; 0.50]*100;
du_min = -du_max;

% Wheel speed limits [rad/s]
Omega_max = RW_max_speed * ones(4,1);
Omega_min = -Omega_max;

%% dumping reference
% % saturation ratio
% sat_ratio = max(abs(Omega_rw) ./ (Omega_max + 1e-12));
% 
% % activation factor alpha
% if sat_ratio <= sat_start
%     alpha = 0.0;
% else
%     alpha = (sat_ratio - sat_start) / (1.0 - sat_start);
%     if alpha > 1.0
%         alpha = 1.0;
%     end
% end
alpha =  0;
tau_dump_ref = -alpha * As * Iws * (Omega_rw - Omega_ref);

% % approximate RCS torque clipping
% for i = 1:3
%     if tau_dump_ref(i) > tau_rcs_max(i)
%         tau_dump_ref(i) = tau_rcs_max(i);
%     elseif tau_dump_ref(i) < -tau_rcs_max(i)
%         tau_dump_ref(i) = -tau_rcs_max(i);
%     end
% end

%% decision variable
% z = [u_rw(4); tau_rcs(3); s1(3); s2(3)]  => total 13

%% cost

Wu   = eye(4);
Wrcs = eta_rcs * eye(3);
V1   = v1      * eye(3);
V2   = v2      * eye(3);

H = blkdiag(Wu, Wrcs, V1, V2);
H = 0.5*(H + H') + 1e-9*eye(13);

f = zeros(13,1);

%% equality constraints
% 1) attitude torque:
%    -As*u_rw + tau_rcs - s1 = tau_pd
%
% 2) dumping torque:
%    tau_rcs - s2 = tau_dump_ref

Aeq = [       -As, eye(3),     -eye(3), zeros(3,3);
       zeros(3,4), eye(3),  zeros(3,3),    -eye(3)];

beq = [      tau_pd;
       tau_dump_ref];

%% bounds
% RW torque bounds
% Torque-rate bounds
lb_rate = u_prev(1:4) + du_min * dt;
ub_rate = u_prev(1:4) + du_max * dt;

% Speed-next bounds
% Omega_next = Omega_rw + dt*(u./Jw)
% => u >= Jw .* (Omega_min - Omega_rw)/dt
% => u <= Jw .* (Omega_max - Omega_rw)/dt
lb_speed = diag(Iws) .* ((Omega_min - Omega_rw) / dt);
ub_speed = diag(Iws) .* ((Omega_max - Omega_rw) / dt);

% Final bounds
lb_u = inf*max(u_rw_min, max(lb_rate, lb_speed));
ub_u = min(u_rw_max, min(ub_rate, ub_speed));

% Feasibility repair
% for i = 1:4
%     if lb_u(i) > ub_u(i)
%         c = 0.5 * (lb_u(i) + ub_u(i));
%         lb_u(i) = c;
%         ub_u(i) = c;
%     end
% end


% RCS torque bounds
% lb_t = -tau_rcs_max;
% ub_t =  tau_rcs_max;
lb_t = -inf*ones(3,1);
ub_t =  inf*ones(3,1);

% slack bounds
big = 1e6;  % inf
lb_s1 = -big * ones(3,1);
ub_s1 =  big * ones(3,1);
lb_s2 = -big * ones(3,1);
ub_s2 =  big * ones(3,1);

lb = [lb_u; lb_t; lb_s1; lb_s2];
ub = [ub_u; ub_t; ub_s1; ub_s2];

%% initial guess
x0 = [zeros(4,1);
      zeros(3,1);
      -tau_pd;
      -tau_dump_ref];
% rw : Omegad cmd, rcs : tau cmd, 
% x0 = min(max(u_prev, lb), ub);

%% solve
options = optimoptions('quadprog', ...
    'Algorithm', 'active-set', ...
    'Display', 'off', ...
    'ConstraintTolerance', 1e-6, ...
    'OptimalityTolerance', 1e-6, ...
    'StepTolerance', 1e-12, ...
    'MaxIterations', 50);

[z, ~, exitflag] = quadprog(H, f, [], [], Aeq, beq, lb, ub, x0, options);

if isempty(z) || exitflag <= 0
    z = x0;
end

%% outputs
u_rw_cmd    = z(1:4);
tau_rcs_cmd = z(5:7);
s1          = z(8:10);
s2          = z(11:13);

tau_rw_body = -As * u_rw_cmd;
% tau_total   = tau_rw_body + tau_rcs_cmd;
u_save = z;
exitflag_out = exitflag;
end
